simulink model "ControladorPI"  (R2018a)
settings: Solver=VariableStepAuto  StartTime=0.0  StopTime=20.0  RelTol=1e-3
values from neighbouring files (symbols this model uses):
  C = GYzss.C    [ProjetoControlPI.m]    (also in ident.m)
  F = FKi(1:size(G,2))    [ProjetoControlPI.m]    (also in ident.m = acker(G, H, P))
  G = GYzss.A    [ProjetoControlPI.m]    (also in ident.m)
  H = GYzss.B    [ProjetoControlPI.m]    (also in ident.m)
  Kc = 1/Y(end)    [ProjetoControlPI.m]    (also in ident.m = dcgain(SysCtl))
  Ki = FKi(size(G,2)+1:end)    [ProjetoControlPI.m]
  L = L'    [ProjetoControlPI.m]    (also in ident.m)
  Ts = 0.001*fd    (= 0.013)    [ProjetoControlPI.m]    (also in ident.m = 0.1)
settings Model: Creator=castr  LastModifiedBy=dougl

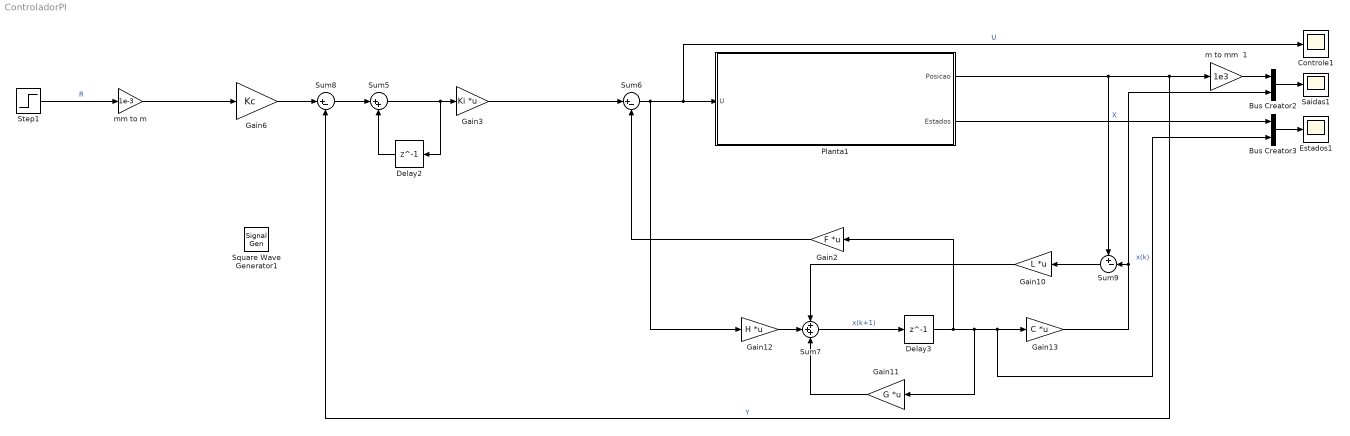
== system ControladorPI ==
  Bus Creator2 : BusCreator  Inputs=2
  Bus Creator3 : BusCreator  Inputs=2
  Controle1 : Scope
  Delay2 : Delay  DelayLength=1
  Delay3 : Delay  DelayLength=1  SampleTime=Ts
  Estados1 : Scope
  Gain10 : Gain  Gain=L  Multiplication=Matrix(K*u)
  Gain11 : Gain  Gain=G  Multiplication=Matrix(K*u)
  Gain12 : Gain  Gain=H  Multiplication=Matrix(K*u)
  Gain13 : Gain  Gain=C  Multiplication=Matrix(K*u)
  Gain2 : Gain  Gain=F  Multiplication=Matrix(K*u)
  Gain3 : Gain  Gain=Ki  Multiplication=Matrix(K*u)
  Gain6 : Gain  Gain=Kc
  Planta1 : Subsystem
  Saidas1 : Scope
  Square Wave Generator1 : SignalGenerator  WaveForm=square  Units=rad/sec
  Step1 : Step  SampleTime=0
  Sum5 : Sum  Inputs=|++
  Sum6 : Sum  Inputs=|+-
  Sum7 : Sum  Inputs=+++
  Sum8 : Sum  Inputs=|+-
  Sum9 : Sum  Inputs=+-|
  m to mm  1 : Gain  Gain=1e3  SaturateOnIntegerOverflow=on  OutDataTypeStr=Inherit: Same as input  ParamDataTypeStr=Inherit: Same as input
  mm to m : Gain  Gain=1e-3
  wires:
  Step1/1 -> mm to m/1  "R"
  Bus Creator2/1 -> Saidas1/1
  Gain11/1 -> Sum7/3
  Sum7/1 -> Delay3/1  "x(k+1)"
  Gain10/1 -> Sum7/1
  Planta1/2(Estados) -> Bus Creator3/1  "X"
  Planta1/1(Posicao) -> m to mm  1/1, Sum8/2, Sum9/1  "Y"
  Bus Creator3/1 -> Estados1/1
  Sum6/1 -> Gain12/1, Controle1/1, Planta1/1(U)  "U"
  Delay3/1 -> Gain2/1, Gain13/1, Bus Creator3/2, Gain11/1  "x(k)"
  Gain12/1 -> Sum7/2
  Delay2/1 -> Sum5/2
  Gain13/1 -> Sum9/2, Bus Creator2/2
  Sum9/1 -> Gain10/1
  Gain2/1 -> Sum6/2
  Sum8/1 -> Sum5/1
  Sum5/1 -> Delay2/1, Gain3/1
  Gain6/1 -> Sum8/1
  Gain3/1 -> Sum6/1
  mm to m/1 -> Gain6/1
  m to mm  1/1 -> Bus Creator2/1

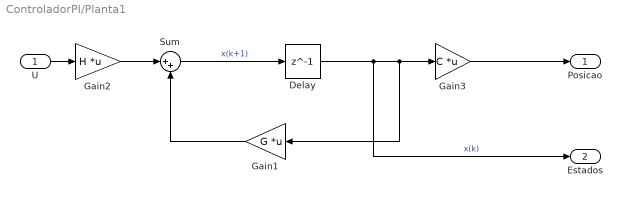
== system ControladorPI/Planta1 ==
  U : Inport
  Delay : Delay  DelayLength=1  InitialCondition=[0 0]  SampleTime=Ts
  Gain1 : Gain  Gain=G  Multiplication=Matrix(K*u)
  Gain2 : Gain  Gain=H  Multiplication=Matrix(K*u)
  Gain3 : Gain  Gain=C  Multiplication=Matrix(K*u)
  Sum : Sum  Inputs=|++
  Posicao : Outport
  Estados : Outport  Port=2
  wires:
  Gain1/1 -> Sum/2
  Gain2/1 -> Sum/1
  U/1 -> Gain2/1
  Sum/1 -> Delay/1  "x(k+1)"
  Delay/1 -> Estados/1, Gain1/1, Gain3/1  "x(k)"
  Gain3/1 -> Posicao/1
